simulink model "test_model"  (R2023b)
settings: Solver=VariableStepAuto  StartTime=0.0  StopTime=inf  RelTol=1e-3
undefined symbols (not defined in the file or in its folder): avoidance_test
libraries: vrlib x1
settings Model: Creator=hampek  LastModifiedBy=hampek

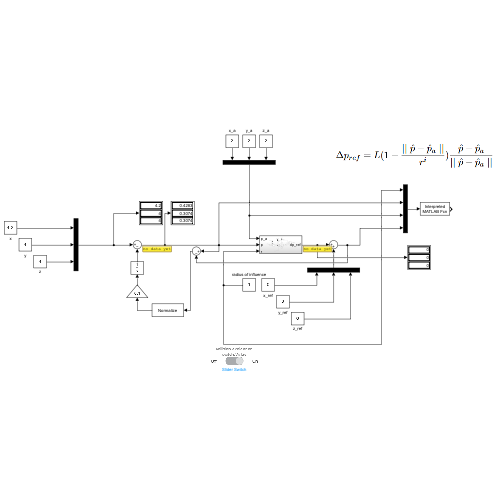
[thumbnail: Simulink's stored preview of the top-level diagram]
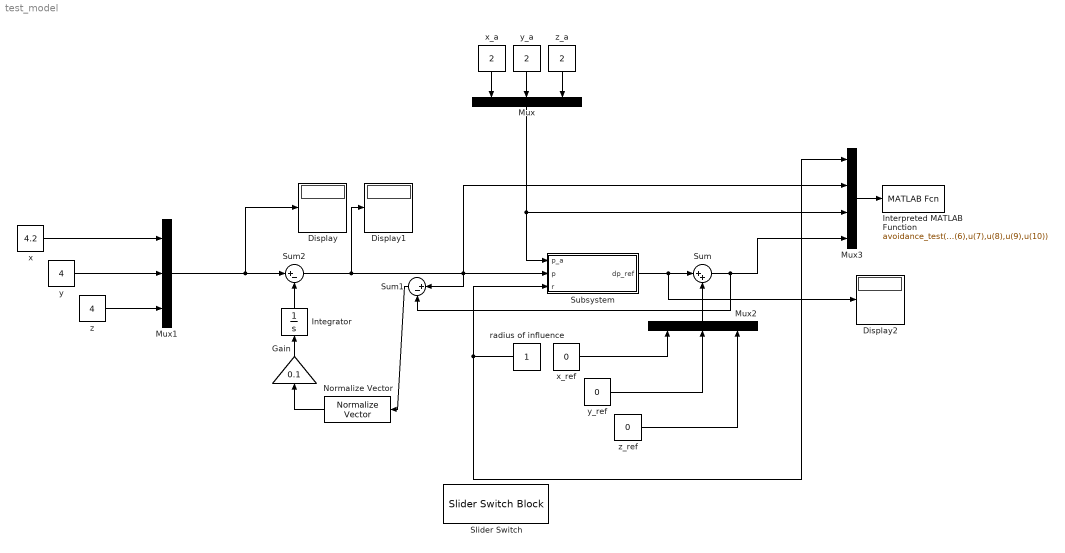
== system test_model ==
  Display : Display
  Display1 : Display
  Display2 : Display
  Gain : Gain  Gain=0.1
  Integrator : Integrator
  Interpreted MATLAB Function : MATLABFcn  MATLABFcn=avoidance_test(u(1),u(2),u(3),u(4),u(5),u(6),u(7),u(8),u(9),u(10))
  Mux : Mux  Inputs=3
  Mux1 : Mux  Inputs=3
  Mux2 : Mux  Inputs=3
  Mux3 : Mux
  Normalize Vector : vrlib/Utilities/Normalize Vector  maxzero=0
  Slider Switch : SliderSwitchBlock
      settings: Values={{'Off', 'On'}, [1 0]}
  Subsystem : Subsystem
  Sum : Sum  Inputs=|++
  Sum1 : Sum  Inputs=|+-
  Sum2 : Sum  Inputs=|+-
  radius of influence : Constant
  x : Constant  Value=4.2
  x_a : Constant  Value=2
  x_ref : Constant  Value=0
  y : Constant  Value=4
  y_a : Constant  Value=2
  y_ref : Constant  Value=0
  z : Constant  Value=4
  z_a : Constant  Value=2
  z_ref : Constant  Value=0
  wires:
  z_a/1 -> Mux/3
  y_a/1 -> Mux/2
  x_a/1 -> Mux/1
  y/1 -> Mux1/2
  x/1 -> Mux1/1
  z/1 -> Mux1/3
  Mux/1 -> Mux3/3, Subsystem/1(p_a)
  radius of influence/1 -> Subsystem/3(r), Mux3/1
  x_ref/1 -> Mux2/1
  y_ref/1 -> Mux2/2
  z_ref/1 -> Mux2/3
  Subsystem/1(dp_ref) -> Display2/1, Sum/1
  Mux2/1 -> Sum/2
  Sum/1 -> Sum1/2, Mux3/4
  Mux3/1 -> Interpreted MATLAB Function/1
  Sum1/1 -> Normalize Vector/1
  Mux1/1 -> Display/1, Sum2/1
  Sum2/1 -> Display1/1, Mux3/2, Sum1/1, Subsystem/2(p)
  Normalize Vector/1 -> Gain/1
  Gain/1 -> Integrator/1
  Integrator/1 -> Sum2/2

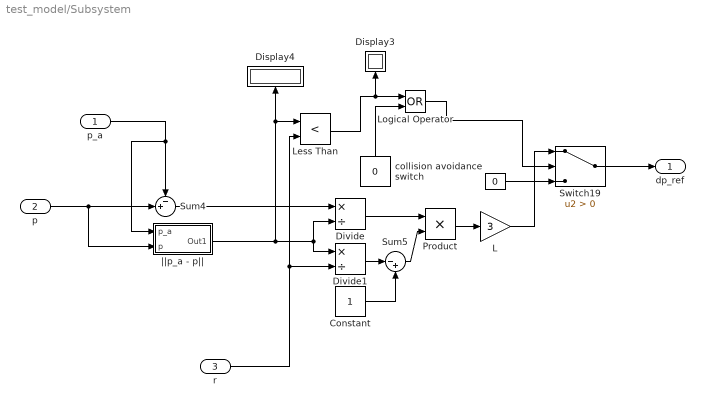
== system test_model/Subsystem ==
  p_a : Inport
  p : Inport  Port=2
  r : Inport  Port=3
  " " : Constant  Value=0
  Constant : Constant
  Display3 : Display
  Display4 : Display
  Divide : Product  Inputs=*/
  Divide1 : Product  Inputs=*/
  L : Gain  Gain=3
  Less Than : RelationalOperator  Operator=<  OutDataTypeStr=boolean  RndMeth=Simplest  InputSameDT=off
  Logical Operator : Logic  Operator=OR  AllPortsSameDT=off  OutDataTypeStr=boolean
  Product : Product
  Sum4 : Sum  Inputs=-+|
  Sum5 : Sum  Inputs=|-+
  Switch19 : Switch  Criteria=u2 > Threshold  SaturateOnIntegerOverflow=off  InputSameDT=off
  collision avoidance switch : Constant  Value=0
  ||p_a - p|| : Subsystem
  dp_ref : Outport
  wires:
  r/1 -> Less Than/2, Divide1/2
  ||p_a - p||/1(Out1) -> Less Than/1, Display4/1, Divide1/1, Divide/2
  p_a/1 -> Sum4/1, ||p_a - p||/1(p_a)
  Divide1/1 -> Sum5/1
  Constant/1 -> Sum5/2
  Sum4/1 -> Divide/1
  Sum5/1 -> Product/2
  " "/1 -> Switch19/3
  Divide/1 -> Product/1
  collision avoidance switch/1 -> Logical Operator/2
  Less Than/1 -> Logical Operator/1, Display3/1
  L/1 -> Switch19/1
  Switch19/1 -> dp_ref/1
  Logical Operator/1 -> Switch19/2
  Product/1 -> L/1
  p/1 -> Sum4/2, ||p_a - p||/2(p)

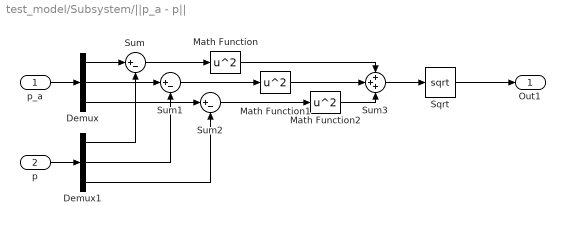
== system test_model/Subsystem/||p_a - p|| ==
  p_a : Inport
  p : Inport  Port=2
  Demux : Demux  Outputs=3
  Demux1 : Demux  Outputs=3
  Math Function : Math  Operator=square
  Math Function1 : Math  Operator=square
  Math Function2 : Math  Operator=square
  Sqrt : Sqrt
  Sum : Sum  Inputs=|+-
  Sum1 : Sum  Inputs=|+-
  Sum2 : Sum  Inputs=|+-
  Sum3 : Sum  Inputs=+++
  Out1 : Outport
  wires:
  p_a/1 -> Demux/1
  p/1 -> Demux1/1
  Demux/3 -> Sum2/1
  Demux/1 -> Sum/1
  Demux/2 -> Sum1/1
  Demux1/1 -> Sum/2
  Demux1/2 -> Sum1/2
  Demux1/3 -> Sum2/2
  Sum/1 -> Math Function/1
  Sum1/1 -> Math Function1/1
  Sum2/1 -> Math Function2/1
  Math Function1/1 -> Sum3/2
  Math Function2/1 -> Sum3/3
  Math Function/1 -> Sum3/1
  Sum3/1 -> Sqrt/1
  Sqrt/1 -> Out1/1
